simulink library "powerlib_extras"  (Simulink 6.0)
settings: Solver=ode45  SolverMode=SingleTasking  StartTime=0.0  StopTime=10.0  RelTol=1e-3
values from neighbouring files (symbols this model uses):
  Ts = get(handles.edit1,'string')    [powergui.m]
undefined symbols (not defined in the file or in its folder): Ac, Bc, Cc, Dc, Delay_discrete, dend, DiscIntNeverNeededParam, extra_sc, j, numd, test_alpha
libraries: powerlib2 x112, powerlib_extras x70, simulink_extras x25, simulink x12, powerlib_models x8
(part 4 of 9)

== system powerlib_extras/Control  Blocks/PWM Generator ==
  note: Pierre Giroux, Gilbert Sybille
      | Power System Laboratory, IREQ
      | Hydro-Quebec
  note: PWM Generator
  Signal(s) : Inport  Port=1  PortDimensions=Signal_PortWidth  LatchInput=off
  BL4 : Logic  Operator=NOT  Inputs=1
  BL5 : Logic  Operator=NOT  Inputs=1
  Constant : Constant  Value=Internal_Phase
  Constant1 : Constant  Value=Internal
  Data Type  Conversion : DataTypeConversion  Orientation=down  OutDataTypeMode=double  SaturateOnIntegerOverflow=on  RndMeth=Zero
  Data Type  Conversion1 : DataTypeConversion  OutDataTypeMode=boolean  SaturateOnIntegerOverflow=on  RndMeth=Zero
  Data Type  Conversion2 : DataTypeConversion  OutDataTypeMode=boolean  SaturateOnIntegerOverflow=on  RndMeth=Zero
  Gain : Gain  Gain=2*pi*Freq  SaturateOnIntegerOverflow=on
  Gain2 : Gain  Gain=pi/180  SaturateOnIntegerOverflow=on
  Gain3 : Gain  Gain=-1  SaturateOnIntegerOverflow=on
  Mux : Mux  Inputs=2
  Mux1 : Mux  Inputs=2
  Mux2 : Mux  Inputs=2
  Product : Product  SaturateOnIntegerOverflow=on  InputSameDT=on
  Relational Operator : RelationalOperator  InputSameDT=on
  Relational Operator1 : RelationalOperator  InputSameDT=on
  Select1A : Selector  Elements=Select1_Elements  InputPortWidth=Select1_PortWidth
  Select1B : Selector  Elements=Select1_Elements  InputPortWidth=Select1_PortWidth
  Select3 : Selector  Elements=Select3_Elements  InputPortWidth=Select3_PortWidth
  Sum : Sum  Inputs=+++  SaturateOnIntegerOverflow=on  InputSameDT=on
  Switch : Switch  Threshold=0.5  InputSameDT=on
  Triangle : simulink/Sources/Repeating Sequence  rep_seq_t=[0 1/Fc/4 3/Fc/4 1/Fc]  rep_seq_y=[0 -1 1 0]
  Trigonometric Function : Trigonometry
  m3 : Constant  Value=Phase
  m4 : Constant  Value=mIndex
  t : Clock
      settings: Decimation=10
  Pulses : Outport
  wires:
  Triangle/1 -> Relational Operator/2, Relational Operator1/2
  Switch/1 -> Relational Operator/1, Gain3/1
  Mux2/1 -> Select3/1
  Select1B/1 -> Mux2/2
  Select1A/1 -> Mux2/1
  Mux1/1 -> Select1B/1
  Mux/1 -> Select1A/1
  BL5/1 -> Mux1/2
  BL4/1 -> Mux/2
  Gain3/1 -> Relational Operator1/1
  Product/1 -> Switch/1
  Constant1/1 -> Switch/2
  Signal(s)/1 -> Switch/3
  Trigonometric Function/1 -> Product/2
  Sum/1 -> Trigonometric Function/1
  m4/1 -> Product/1
  Constant/1 -> Sum/3
  m3/1 -> Gain2/1
  Gain2/1 -> Sum/2
  Gain/1 -> Sum/1
  t/1 -> Gain/1
  Select3/1 -> Data Type  Conversion/1
  Data Type  Conversion/1 -> Pulses/1
  Relational Operator/1 -> Data Type  Conversion1/1
  Data Type  Conversion1/1 -> BL4/1, Mux/1
  Relational Operator1/1 -> Data Type  Conversion2/1
  Data Type  Conversion2/1 -> BL5/1, Mux1/1

== system powerlib_extras/Control  Blocks/Sample & Hold ==
  note: Sample and Hold
  note: Silvano Casoria
      | Power System Simulation Laboratory
      | IREQ, Hydro-Quebc
  In : Inport  Port=1  LatchInput=off
  S : Inport  Port=2  LatchInput=off
  IC=ic : Memory  Orientation=left  X0=ic  InheritSampleTime=on
  Switch : Switch  Threshold=0.5  SaturateOnIntegerOverflow=on  InputSameDT=on
  "   " : Outport  InitialOutput=0
  wires:
  Switch/1 -> "   "/1, IC=ic/1
  IC=ic/1 -> Switch/3
  In/1 -> Switch/1
  S/1 -> Switch/2

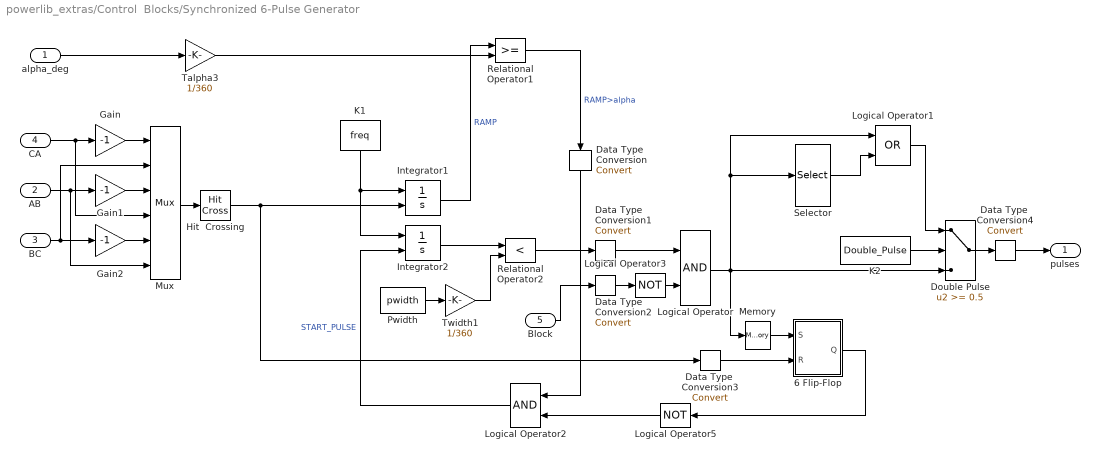
== system powerlib_extras/Control  Blocks/Synchronized 6-Pulse Generator ==
  alpha_deg : Inport  Port=1  LatchInput=off
  AB : Inport  Port=2  LatchInput=off
  BC : Inport  Port=3  LatchInput=off
  CA : Inport  Port=4  LatchInput=off
  Block : Inport  Port=5  LatchInput=off
  6 Flip-Flop : Subsystem
  Data Type  Conversion : DataTypeConversion  Orientation=down  OutDataTypeMode=boolean  SaturateOnIntegerOverflow=on  RndMeth=Zero
  Data Type  Conversion1 : DataTypeConversion  OutDataTypeMode=boolean  SaturateOnIntegerOverflow=on  RndMeth=Zero
  Data Type  Conversion2 : DataTypeConversion  OutDataTypeMode=boolean  SaturateOnIntegerOverflow=on  RndMeth=Zero
  Data Type  Conversion3 : DataTypeConversion  OutDataTypeMode=boolean  SaturateOnIntegerOverflow=on  RndMeth=Zero
  Data Type  Conversion4 : DataTypeConversion  OutDataTypeMode=double  SaturateOnIntegerOverflow=on  RndMeth=Zero
  Double Pulse : Switch  Threshold=0.5  InputSameDT=on
  Gain : Gain  Gain=-1  SaturateOnIntegerOverflow=on
  Gain1 : Gain  Gain=-1  SaturateOnIntegerOverflow=on
  Gain2 : Gain  Gain=-1  SaturateOnIntegerOverflow=on
  Hit  Crossing : HitCross  HitCrossingDirection=rising
  Integrator1 : Integrator  ExternalReset=rising
  Integrator2 : Integrator  ExternalReset=rising
  K1 : Constant  Orientation=down  Value=freq
  K2 : Constant  Value=Double_Pulse
  Logical Operator : Logic
  Logical Operator1 : Logic  Operator=OR
  Logical Operator2 : Logic  Orientation=left
  Logical Operator3 : Logic  Operator=NOT  Inputs=1
  Logical Operator5 : Logic  Orientation=left  Operator=NOT  Inputs=1
  Memory : Memory
  Mux : Mux  Inputs=6
  Pwidth : Constant  Value=pwidth
  Relational Operator1 : RelationalOperator  InputSameDT=on
  Relational Operator2 : RelationalOperator  Operator=<  InputSameDT=on
  Selector : Selector  Elements=[2 3 4 5 6 1 ]  InputPortWidth=6
  Talpha3 : Gain  Gain=1/360  SaturateOnIntegerOverflow=on
  Twidth1 : Gain  Gain=1/360  SaturateOnIntegerOverflow=on
  pulses : Outport  InitialOutput=0
  wires:
  alpha_deg/1 -> Talpha3/1
  Gain/1 -> Mux/1
  Gain1/1 -> Mux/3
  Gain2/1 -> Mux/5
  BC/1 -> Gain2/1, Mux/2
  CA/1 -> Gain/1, Mux/4
  AB/1 -> Gain1/1, Mux/6
  Mux/1 -> Hit  Crossing/1
  K1/1 -> Integrator1/1, Integrator2/1
  Pwidth/1 -> Twidth1/1
  Hit  Crossing/1 -> Integrator1/2, Data Type  Conversion3/1
  Logical Operator5/1 -> Logical Operator2/2
  Logical Operator2/1 -> Integrator2/2  "START_PULSE"
  6 Flip-Flop/1(Q) -> Logical Operator5/1
  Logical Operator3/1 -> Logical Operator/2
  Twidth1/1 -> Relational Operator2/2
  Integrator2/1 -> Relational Operator2/1
  Talpha3/1 -> Relational Operator1/2
  Integrator1/1 -> Relational Operator1/1  "RAMP"
  Memory/1 -> 6 Flip-Flop/1(S)
  K2/1 -> Double Pulse/2
  Logical Operator/1 -> Memory/1, Selector/1, Logical Operator1/1, Double Pulse/3
  Selector/1 -> Logical Operator1/2
  Relational Operator1/1 -> Data Type  Conversion/1  "RAMP>alpha"
  Data Type  Conversion/1 -> Logical Operator2/1
  Relational Operator2/1 -> Data Type  Conversion1/1
  Data Type  Conversion1/1 -> Logical Operator/1
  Block/1 -> Data Type  Conversion2/1
  Data Type  Conversion2/1 -> Logical Operator3/1
  Data Type  Conversion3/1 -> 6 Flip-Flop/2(R)
  Logical Operator1/1 -> Double Pulse/1
  Double Pulse/1 -> Data Type  Conversion4/1
  Data Type  Conversion4/1 -> pulses/1

== system powerlib_extras/Control  Blocks/Timer ==
  Clock : Clock
      settings: Decimation=10
  Derivative : Derivative
  Hit  Crossing : HitCross  ShowOutputPort=off
  Look-Up Table : Lookup  DialogController=Simulink.DDGSource  InputValues=tv  OutputValues=opv  SaturateOnIntegerOverflow=on
  Out : Outport
  wires:
  Derivative/1 -> Hit  Crossing/1
  Look-Up Table/1 -> Derivative/1, Out/1
  Clock/1 -> Look-Up Table/1

== system powerlib_extras/Discrete Measurements/Discrete PLL-Driven  Fundamental Value ==
  note: Pierre Giroux, Gilbert Sybille
      | Power System Simulation Laboratory
      | IREQ, Hydro-Quebc
  note: Discrete PLL-Driven Fundamental Value
  Freq : Inport  Port=1  LatchInput=off
  Sin_Cos : Inport  Port=2  PortDimensions=2  LatchInput=off
  In : Inport  Port=3  LatchInput=off
  Cartesian to Polar : simulink_extras/Transformations/Cartesian to Polar
  Demux : Demux  Outputs=2
  Discrete Variable Frequency Mean value : powerlib_extras/Discrete Measurements/Discrete Variable Frequency Mean value  Finit=Finit  Fmin=Fmin  Vinit=Real_Init  Ts=Ts
  Discrete Variable Frequency Mean value1 : powerlib_extras/Discrete Measurements/Discrete Variable Frequency Mean value  Finit=Finit  Fmin=Fmin  Vinit=Imag_Init  Ts=Ts
  Gain1 : Gain  Gain=2  SaturateOnIntegerOverflow=on
  Product : Product  SaturateOnIntegerOverflow=on  InputSameDT=on
  Rad->Deg. : Gain  Gain=180/pi  SaturateOnIntegerOverflow=on
  Mag : Outport
  Phase : Outport  Port=2
  wires:
  In/1 -> Product/1
  Sin_Cos/1 -> Gain1/1
  Freq/1 -> Discrete Variable Frequency Mean value/1, Discrete Variable Frequency Mean value1/1
  Demux/2 -> Discrete Variable Frequency Mean value1/2
  Product/1 -> Demux/1
  Gain1/1 -> Product/2
  Demux/1 -> Discrete Variable Frequency Mean value/2
  Rad->Deg./1 -> Phase/1
  Cartesian to Polar/1 -> Mag/1
  Cartesian to Polar/2 -> Rad->Deg./1
  Discrete Variable Frequency Mean value/1 -> Cartesian to Polar/1  "Real"
  Discrete Variable Frequency Mean value1/1 -> Cartesian to Polar/2  "Imag"

== system powerlib_extras/Discrete Measurements/Discrete Variable Frequency Mean value ==
  note: Variable frequency - Discrete Mean Value
  note: Pierre Giroux, Gilbert Sybille, Richard Gagnon
      | Power System Simulation Laboratory
      | IREQ, Hydro-Quebc
  note: link disabled
  Freq : Inport  Port=1  PortDimensions=1  LatchInput=off
  In : Inport  Port=2  PortDimensions=1  LatchInput=off
  Constant : Constant  Value=Vinit
  Correction subsystem : Subsystem
  Discrete Variable Transport Delay : Subsystem  AncestorBlock=|  mask(Discrete variable transport delay){MaxDelay=MaxDelay, InitialValue=0, Ts=Ts}
      | powerlib_extras/Discrete 
      | Control Blocks/Discrete Variable
      | Transport Delay
      mask prompts: MaxDelay "Maximum delay (s):"; InitialValue "Initial input:"; Ts "Sample time:"
      mask help:
      | Apply a delay to the first input (In) signal.
      | The second input (D) specifies the delay time.
  Gain : Gain  Gain=Ts  SaturateOnIntegerOverflow=on
  Integ4 : DiscreteIntegrator  IntegratorMethod=Integration: Trapezoidal  SampleTime=Ts  ICPrevOutput=DiscIntNeverNeededParam  ICPrevScaledInput=DiscIntNeverNeededParam
  Number of samples per cycle : Fcn  Expr=1/u[1]/Ts
  Product : Product  SaturateOnIntegerOverflow=on  InputSameDT=on
  Rounding Function : Rounding  Operator=ceil
  Step : Step  Time=1/Finit  SampleTime=Ts
  Sum5 : Sum  SaturateOnIntegerOverflow=on  InputSameDT=on
  Sum7 : Sum  Inputs=-+  SaturateOnIntegerOverflow=on  InputSameDT=on
  Switch : Switch  Threshold=0.5  InputSameDT=on
  To avoid division by zero : Saturate  Orientation=down  UpperLimit=1e6  LowerLimit=1e-6
  Mean : Outport
  wires:
  Step/1 -> Switch/2
  Correction subsystem/1(Out) -> Sum5/2
  To avoid division by zero/1 -> Number of samples per cycle/1  "Freq"
  Switch/1 -> Mean/1
  Constant/1 -> Switch/3
  Sum5/1 -> Switch/1
  Number of samples per cycle/1 -> Correction subsystem/1(N), Rounding Function/1
  Rounding Function/1 -> Correction subsystem/2(F), Gain/1
  Gain/1 -> Discrete Variable Transport Delay/2(D)  "Delay"
  Freq/1 -> To avoid division by zero/1, Product/2  "Freq"
  Integ4/1 -> Sum7/2, Discrete Variable Transport Delay/1(In)
  Sum7/1 -> Product/1
  Discrete Variable Transport Delay/1(Out) -> Sum7/1
  Product/1 -> Sum5/1  "Mean value"
  In/1 -> Correction subsystem/3(In), Integ4/1  "In"

== system powerlib_extras/Discrete Measurements/Discrete  Active  & Reactive  Power ==
  note: Pierre Giroux, Gilbert Sybille
      | Power System Simulation Laboratory
      | IREQ, Hydro-Quebc
  note: Discrete Active & Reactive Power at fundamental frequency
  V : Inport  Port=1  LatchInput=off
  I : Inport  Port=2  LatchInput=off
  Deg->Rad : Gain  Gain=pi/180  SaturateOnIntegerOverflow=on
  Discrete  I_Fundamental : powerlib_extras/Discrete Measurements/Discrete  Fourier  Freq=Freq  n=1  Par_Init=Par_Iinit  Ts=Ts
  Discrete  V_Fundamental : powerlib_extras/Discrete Measurements/Discrete  Fourier  Freq=Freq  n=1  Par_Init=Par_Vinit  Ts=Ts
  Gain : Gain  Gain=1/2  SaturateOnIntegerOverflow=on
  Mux : Mux  Inputs=2
  Mux1 : Mux  Inputs=2
  Product : Product  SaturateOnIntegerOverflow=on  InputSameDT=on
  Product1 : Product  SaturateOnIntegerOverflow=on  InputSameDT=on
  Product2 : Product  SaturateOnIntegerOverflow=on  InputSameDT=on
  Sum : Sum  Inputs=+-  SaturateOnIntegerOverflow=on  InputSameDT=on
  Trigonometric Function : Trigonometry
  Trigonometric Function1 : Trigonometry  Operator=cos
  Mag_V_I : Outport
  P_Q : Outport  Port=2
  wires:
  V/1 -> Discrete  V_Fundamental/1
  I/1 -> Discrete  I_Fundamental/1
  Discrete  V_Fundamental/2 -> Sum/1
  Discrete  I_Fundamental/2 -> Sum/2
  Sum/1 -> Deg->Rad/1
  Deg->Rad/1 -> Trigonometric Function1/1, Trigonometric Function/1
  Trigonometric Function/1 -> Product2/2
  Product/1 -> Product1/1, Product2/1
  Trigonometric Function1/1 -> Product1/2
  Mux/1 -> Mag_V_I/1
  Discrete  V_Fundamental/1 -> Product/1, Mux/1
  Discrete  I_Fundamental/1 -> Product/2, Mux/2
  Product1/1 -> Mux1/1
  Product2/1 -> Mux1/2
  Mux1/1 -> Gain/1
  Gain/1 -> P_Q/1

== system powerlib_extras/Discrete Measurements/Discrete  Fourier ==
  note: Discrete Fourier
  note: Pierre Giroux, Gilbert Sybille
      | Power System Simulation Laboratory
      | IREQ, Hydro-Quebc
  In : Inport  Port=1  LatchInput=off
  Cartesian to Polar : simulink_extras/Transformations/Cartesian to Polar
  Demux : Demux  Outputs=2
  Discrete  Mean value1 : powerlib_extras/Discrete Measurements/Discrete  Mean value  Freq=Freq  Vinit=Real_Init  Ts=Ts
  Discrete  Mean value2 : powerlib_extras/Discrete Measurements/Discrete  Mean value  Freq=Freq  Vinit=Imag_Init  Ts=Ts
  Gain : Gain  Gain=2*pi*n*Freq  SaturateOnIntegerOverflow=on
  Gain1 : Gain  Gain=k  SaturateOnIntegerOverflow=on
  Mux : Mux  Inputs=2
  Product : Product  SaturateOnIntegerOverflow=on  InputSameDT=on
  Rad->Deg. : Gain  Gain=180/pi  SaturateOnIntegerOverflow=on
  Trigonometric Function : Trigonometry
  Trigonometric Function1 : Trigonometry  Operator=cos
  t : DigitalClock  SampleTime=Ts
  Mag : Outport
  Phase : Outport  Port=2
  wires:
  t/1 -> Gain/1
  Gain/1 -> Trigonometric Function/1, Trigonometric Function1/1
  Trigonometric Function/1 -> Mux/1
  Trigonometric Function1/1 -> Mux/2
  Mux/1 -> Gain1/1
  In/1 -> Product/1
  Gain1/1 -> Product/2
  Product/1 -> Demux/1
  Demux/1 -> Discrete  Mean value1/1
  Demux/2 -> Discrete  Mean value2/1
  Discrete  Mean value1/1 -> Cartesian to Polar/1  "Real"
  Discrete  Mean value2/1 -> Cartesian to Polar/2  "Imag"
  Cartesian to Polar/2 -> Rad->Deg./1
  Cartesian to Polar/1 -> Mag/1
  Rad->Deg./1 -> Phase/1

== system powerlib_extras/Discrete Measurements/Discrete  Mean value ==
  note: Discrete Mean Value
  note: Pierre Giroux, Gilbert Sybille
      | Power System Simulation Laboratory
      | IREQ, Hydro-Quebc
  In : Inport  Port=1  LatchInput=off
  Constant : Constant  Value=Vinit
  Discrete Variable Transport Delay : powerlib_extras/Discrete  Control Blocks/Discrete Variable Transport Delay  MaxDelay=Delay+Ts  InitialValue=0  Ts=Ts
  Gain : Gain  Gain=K1  SaturateOnIntegerOverflow=on
  Gain1 : Gain  Gain=K2  SaturateOnIntegerOverflow=on
  Integ4 : DiscreteIntegrator  IntegratorMethod=Integration: Trapezoidal  SampleTime=Ts  ICPrevOutput=DiscIntNeverNeededParam  ICPrevScaledInput=DiscIntNeverNeededParam
  K1 : Constant  Value=Delay
  K2 : Constant  Value=Freq
  Product : Product  SaturateOnIntegerOverflow=on  InputSameDT=on
  Step : Step  Time=1/Freq  SampleTime=Ts
  Sum1 : Sum  Inputs=+-  SaturateOnIntegerOverflow=on  InputSameDT=on
  Sum5 : Sum  SaturateOnIntegerOverflow=on  InputSameDT=on
  Sum7 : Sum  Inputs=-+  SaturateOnIntegerOverflow=on  InputSameDT=on
  Switch : Switch  Threshold=0.5  InputSameDT=on
  Unit Delay : UnitDelay  SampleTime=Ts
  Mean : Outport
  wires:
  Sum1/1 -> Sum5/2  "Correction"
  Gain/1 -> Sum1/2
  Unit Delay/1 -> Gain/1
  Gain1/1 -> Sum1/1
  K1/1 -> Discrete Variable Transport Delay/2
  Discrete Variable Transport Delay/1 -> Sum7/1
  Switch/1 -> Mean/1
  Constant/1 -> Switch/3
  Step/1 -> Switch/2
  Sum5/1 -> Switch/1
  In/1 -> Unit Delay/1, Gain1/1, Integ4/1  "In"
  K2/1 -> Product/2
  Integ4/1 -> Sum7/2, Discrete Variable Transport Delay/1
  Sum7/1 -> Product/1
  Product/1 -> Sum5/1  "Mean value"

== system powerlib_extras/Discrete Measurements/Discrete  RMS value ==
  note: Gilbert Sybille, Pierre Giroux
      | Power System Simulation Laboratory
      | IREQ, Hydro-Quebc
  note: Discrete RMS value
  In : Inport  Port=1  LatchInput=off
  Discrete  Mean value : powerlib_extras/Discrete Measurements/Discrete  Mean value  Freq=Freq  Vinit=Mag_Init*Mag_Init  Ts=Ts
  Math Function1 : Math  Operator=sqrt  SaturateOnIntegerOverflow=on
  Product : Product  SaturateOnIntegerOverflow=on  InputSameDT=on
  Saturation Ajout P.B pour eviter  sqrt(negatif) : Saturate  UpperLimit=Inf  LowerLimit=0
  RMS : Outport  InitialOutput=0
  wires:
  In/1 -> Product/2, Product/1
  Math Function1/1 -> RMS/1
  Product/1 -> Discrete  Mean value/1
  Discrete  Mean value/1 -> Saturation Ajout P.B pour eviter  sqrt(negatif)/1
  Saturation Ajout P.B pour eviter  sqrt(negatif)/1 -> Math Function1/1

== system powerlib_extras/Discrete Measurements/Discrete  Total  Harmonic Distorsion ==
  note: Pierre Giroux, Gilbert Sybille
      | Power System Simulation Laboratory
      | IREQ, Hydro-Quebc
  note: Discrete Total Harmonic Distortion (THD)
  note: THD= Uhrms /U1rms
  note: Urms = true rms value including harmonics
  note: Uhrms = rms value of harmonics = sqrt( U2^2 + U3^2 + U4^2....) = sqrt( Urms^2 -U1rms^2)
  note: U1rms = rms value of the fundamenrtal component
  note: where:
  note: THD= Uhrms /U1rms
  signal : Inport  Port=1  LatchInput=off
  Constant : Constant  Value=1e-6
  Discrete  Fourier : powerlib_extras/Discrete Measurements/Discrete  Fourier  Freq=Freq  n=1  Par_Init=[0 0]  Ts=Ts
  Discrete  RMS value : powerlib_extras/Discrete Measurements/Discrete  RMS value  Freq=Freq  Mag_Init=0  Ts=Ts
  Math Function2 : Math  Operator=sqrt  SaturateOnIntegerOverflow=on
  Product : Product  Inputs=*/  SaturateOnIntegerOverflow=on  InputSameDT=on
  Product1 : Product  SaturateOnIntegerOverflow=on  InputSameDT=on
  Product2 : Product  SaturateOnIntegerOverflow=on  InputSameDT=on
  Sum : Sum  Inputs=+-  SaturateOnIntegerOverflow=on  InputSameDT=on
  Sum1 : Sum  Inputs=+-  SaturateOnIntegerOverflow=on  InputSameDT=on
  Terminator : Terminator
  peak2rms : Gain  Gain=1/sqrt(2)  SaturateOnIntegerOverflow=on
  THD : Outport
  wires:
  Sum1/1 -> Product/2
  Constant/1 -> Sum1/2
  Discrete  RMS value/1 -> Product1/2, Product1/1  "Urms"
  signal/1 -> Discrete  Fourier/1, Discrete  RMS value/1
  Sum/1 -> Math Function2/1
  Product1/1 -> Sum/1
  Product2/1 -> Sum/2
  Math Function2/1 -> Product/1  "Uhrms"
  Product/1 -> THD/1
  Discrete  Fourier/1 -> peak2rms/1
  peak2rms/1 -> Product2/2, Sum1/1, Product2/1  "U1 rms"
  Discrete  Fourier/2 -> Terminator/1

== system powerlib_extras/Discrete Measurements/Discrete 3-phase PLL-Driven Positive-Sequence Fundamental Value ==
  note: Pierre Giroux, Gilbert Sybille
      | Power System Simulation Laboratory
      | IREQ, Hydro-Quebc
  note: Discrete 3-phase PLL-Driven Positive-Sequence Fundamental Value
  Freq : Inport  Port=1  LatchInput=off
  Sin_Cos : Inport  Port=2  PortDimensions=2  LatchInput=off
  abc : Inport  Port=3  PortDimensions=3  LatchInput=off
  Cartesian to Polar : simulink_extras/Transformations/Cartesian to Polar
  Demux : Demux  Outputs=3
  Discrete Variable Frequency Mean value : powerlib_extras/Discrete Measurements/Discrete Variable Frequency Mean value  Finit=Finit  Fmin=Fmin  Vinit=Real_Init  Ts=Ts
  Discrete Variable Frequency Mean value1 : powerlib_extras/Discrete Measurements/Discrete Variable Frequency Mean value  Finit=Finit  Fmin=Fmin  Vinit=Imag_Init  Ts=Ts
  Rad->Deg. : Gain  Gain=180/pi  SaturateOnIntegerOverflow=on
  Terminator : Terminator
  abc_to_dq0 Transformation : powerlib_extras/Measurements/abc_to_dq0 Transformation
  Mag : Outport
  Phase : Outport  Port=2
  wires:
  Sin_Cos/1 -> abc_to_dq0 Transformation/2
  Freq/1 -> Discrete Variable Frequency Mean value/1, Discrete Variable Frequency Mean value1/1
  Discrete Variable Frequency Mean value/1 -> Cartesian to Polar/1  "Real"
  Rad->Deg./1 -> Phase/1
  Discrete Variable Frequency Mean value1/1 -> Cartesian to Polar/2  "Real"
  Demux/2 -> Discrete Variable Frequency Mean value1/2
  Demux/1 -> Discrete Variable Frequency Mean value/2
  abc/1 -> abc_to_dq0 Transformation/1
  abc_to_dq0 Transformation/1 -> Demux/1
  Demux/3 -> Terminator/1
  Cartesian to Polar/1 -> Mag/1
  Cartesian to Polar/2 -> Rad->Deg./1

== system powerlib_extras/Discrete Measurements/Discrete 3-phase PLL-Driven  Positive-Sequence Active & Reactive Power ==
  note: Pierre Giroux, Gilbert Sybille
      | Power System Simulation Laboratory
      | IREQ, Hydro-Quebc
  note: Discrete 3-phase PLL-driven Positive-Sequence Active & Reactive Power
  Freq : Inport  Port=1  PortDimensions=1  LatchInput=off
  Sin_Cos : Inport  Port=2  PortDimensions=2  LatchInput=off
  Vabc : Inport  Port=3  PortDimensions=3  LatchInput=off
  Iabc : Inport  Port=4  PortDimensions=3  LatchInput=off
  Deg->Rad : Gain  Gain=pi/180  SaturateOnIntegerOverflow=on
  Discrete 3-phase PLL-Driven Positive-Sequence Fundamental Value : powerlib_extras/Discrete Measurements/Discrete 3-phase PLL-Driven Positive-Sequence Fundamental Value  Finit=Finit  Fmin=Fmin  Par_Init=Par_Vinit  Ts=Ts
  Discrete 3-phase PLL-Driven Positive-Sequence Fundamental Value1 : powerlib_extras/Discrete Measurements/Discrete 3-phase PLL-Driven Positive-Sequence Fundamental Value  Finit=Finit  Fmin=Fmin  Par_Init=Par_Iinit  Ts=Ts
  Gain1 : Gain  Gain=3/2  SaturateOnIntegerOverflow=on
  Mux2 : Mux  Inputs=2
  Mux3 : Mux  Inputs=2
  Product : Product  SaturateOnIntegerOverflow=on  InputSameDT=on
  Product1 : Product  SaturateOnIntegerOverflow=on  InputSameDT=on
  Product2 : Product  SaturateOnIntegerOverflow=on  InputSameDT=on
  Sum : Sum  Inputs=+-  SaturateOnIntegerOverflow=on  InputSameDT=on
  Trigonometric Function : Trigonometry
  Trigonometric Function1 : Trigonometry  Operator=cos
  Mag_V_I : Outport
  P_Q : Outport  Port=2
  wires:
  Iabc/1 -> Discrete 3-phase PLL-Driven Positive-Sequence Fundamental Value1/3
  Discrete 3-phase PLL-Driven Positive-Sequence Fundamental Value1/1 -> Product2/2, Mux3/2
  Product2/1 -> Product1/2, Product/1
  Gain1/1 -> P_Q/1
  Mux3/1 -> Mag_V_I/1
  Product1/1 -> Mux2/2
  Product/1 -> Mux2/1
  Mux2/1 -> Gain1/1
  Trigonometric Function/1 -> Product1/1
  Trigonometric Function1/1 -> Product/2
  Deg->Rad/1 -> Trigonometric Function/1, Trigonometric Function1/1
  Sum/1 -> Deg->Rad/1
  Discrete 3-phase PLL-Driven Positive-Sequence Fundamental Value1/2 -> Sum/2
  Discrete 3-phase PLL-Driven Positive-Sequence Fundamental Value/1 -> Product2/1, Mux3/1
  Discrete 3-phase PLL-Driven Positive-Sequence Fundamental Value/2 -> Sum/1
  Sin_Cos/1 -> Discrete 3-phase PLL-Driven Positive-Sequence Fundamental Value/2, Discrete 3-phase PLL-Driven Positive-Sequence Fundamental Value1/2
  Freq/1 -> Discrete 3-phase PLL-Driven Positive-Sequence Fundamental Value/1, Discrete 3-phase PLL-Driven Positive-Sequence Fundamental Value1/1
  Vabc/1 -> Discrete 3-phase PLL-Driven Positive-Sequence Fundamental Value/3

== system powerlib_extras/Discrete Measurements/Discrete 3-phase Positive-Sequence Fundamental Value ==
  note: Discrete Measurement - Positive-sequence Fundamental Value
  note: Pierre Giroux, Gilbert Sybille
      | Power System Simulation Laboratory
      | IREQ, Hydro-Quebc
  abc : Inport  Port=1  PortDimensions=3  LatchInput=off
  Cartesian to Polar : simulink_extras/Transformations/Cartesian to Polar
  Demux : Demux  Outputs=3
  Discrete  Mean value1 : powerlib_extras/Discrete Measurements/Discrete  Mean value  Freq=Freq  Vinit=Real_Init  Ts=Ts
  Discrete  Mean value2 : powerlib_extras/Discrete Measurements/Discrete  Mean value  Freq=Freq  Vinit=Imag_Init  Ts=Ts
  Gain : Gain  Gain=2*pi*Freq  SaturateOnIntegerOverflow=on
  Mux : Mux  Inputs=2
  Rad->Deg. : Gain  Gain=180/pi  SaturateOnIntegerOverflow=on
  Terminator : Terminator
  Trigonometric Function : Trigonometry
  Trigonometric Function1 : Trigonometry  Operator=cos
  abc_to_dq0 Transformation : powerlib_extras/Measurements/abc_to_dq0 Transformation
  t : DigitalClock  SampleTime=Ts
  Mag : Outport
  Phase : Outport  Port=2
  wires:
  Trigonometric Function1/1 -> Mux/2
  Trigonometric Function/1 -> Mux/1
  Demux/1 -> Discrete  Mean value1/1
  Demux/2 -> Discrete  Mean value2/1
  Demux/3 -> Terminator/1
  abc_to_dq0 Transformation/1 -> Demux/1
  Discrete  Mean value2/1 -> Cartesian to Polar/2  "Real"
  Rad->Deg./1 -> Phase/1
  Discrete  Mean value1/1 -> Cartesian to Polar/1  "Real"
  Mux/1 -> abc_to_dq0 Transformation/2
  abc/1 -> abc_to_dq0 Transformation/1
  t/1 -> Gain/1
  Gain/1 -> Trigonometric Function/1, Trigonometric Function1/1
  Cartesian to Polar/1 -> Mag/1
  Cartesian to Polar/2 -> Rad->Deg./1

== system powerlib_extras/Discrete Measurements/Discrete 3-phase Sequence Analyzer ==
  note: Discrete 3-phase Sequence Analyser
  note: Gilbert Sybille, Pierre Giroux
      | Power System Simulation Laboratory
      | IREQ, Hydro-Quebc
  note: Zero sequence :V0 = 1/3 * (Va + Vb + Vc )
  note: where a =exp(j *2pi/3) = 1 < + 120 deg.
  note: Positive sequence :V1 = 1/3 * (Va + a*Vb + a^2 *Vc )
  note: Negative sequence :V2 = 1/3 * (Va + a^2*Vb + a *Vc )
  abc : Inport  Port=1  LatchInput=off
  Complex to Magnitude-Angle : ComplexToMagnitudeAngle
  Constant : Constant  Value=PosOn
  Constant1 : Constant  Value=NegOn
  Constant2 : Constant  Value=ZeroOn
  Demux : Demux  Outputs=3
  Determine if pha20 are set to zero : Subsystem
  "Gain2 " : Gain  Gain=k  SaturateOnIntegerOverflow=on
  Mux : Mux  Inputs=3
  Mux1 : Mux  Inputs=3
  Neg. Seq. Computation : Subsystem  TreatAsAtomicUnit=on
  Phasor A : Subsystem  mask(Discrete Fourier ; Real Imag Outputs){Freq=Freq, Par_Init=[Mag_Init  Phase_Init], Ts=Ts}
      mask prompts: Freq "Fundamental frequency (Hz):"; Par_Init "Initial Input [Mag Phase(degrees)]"; Ts "Sample time:"
      mask init:
      | Real_Init=Par_Init(1)*cos(Par_Init(2)*pi/180);
      | Imag_Init=Par_Init(1)*sin(Par_Init(2)*pi/180);
  Phasor B : powerlib_extras/Discrete Measurements/Discrete 3-phase Sequence Analyzer/Phasor A  Freq=Freq  Par_Init="[Mag_Init  Phase_Init-120]"  Ts=Ts
  Phasor C : powerlib_extras/Discrete Measurements/Discrete 3-phase Sequence Analyzer/Phasor A  Freq=Freq  Par_Init="[Mag_Init  Phase_Init+120]"  Ts=Ts
  Pos. Seq. Computation : Subsystem  TreatAsAtomicUnit=on
  Selector : Selector  Elements=SelectElement  InputPortWidth=3
  Selector1 : Selector  Elements=SelectElement  InputPortWidth=3
  Zero Seq. Computation : Subsystem  TreatAsAtomicUnit=on
  cos(nwt) : Sin  Frequency=2*pi*n*Freq  Phase=pi/2  SampleTime=Ts
  rad->deg1 : Gain  Gain=180/pi  SaturateOnIntegerOverflow=on
  sin(nwt) : Sin  Frequency=2*pi*n*Freq  SampleTime=Ts
  Mag : Outport  InitialOutput=0
  Phase : Outport  Port=2  InitialOutput=0
  wires:
  Phasor C/1 -> Mux/3
  Phasor B/1 -> Mux/2
  Phasor A/1(Out) -> Mux/1
  "Gain2 "/1 -> Demux/1
  abc/1 -> "Gain2 "/1
  Demux/1 -> Phasor A/1(in)
  Demux/2 -> Phasor B/1
  Demux/3 -> Phasor C/1
  sin(nwt)/1 -> Phasor A/2(sin), Phasor B/2, Phasor C/2
  cos(nwt)/1 -> Phasor A/3(cos), Phasor B/3, Phasor C/3
  Mux/1 -> Pos. Seq. Computation/1(In), Neg. Seq. Computation/1(In), Zero Seq. Computation/1(In)
  Pos. Seq. Computation/1(Out) -> Mux1/1
  Neg. Seq. Computation/1(Out) -> Mux1/2
  Zero Seq. Computation/1(Out) -> Mux1/3
  Mux1/1 -> Complex to Magnitude-Angle/1
  Complex to Magnitude-Angle/1 -> Determine if pha20 are set to zero/1(Mag120), Selector/1
  Constant/1 -> Pos. Seq. Computation/Enable
  Constant2/1 -> Zero Seq. Computation/Enable
  Selector/1 -> Mag/1
  Determine if pha20 are set to zero/1(Pha120) -> Selector1/1
  Selector1/1 -> rad->deg1/1
  rad->deg1/1 -> Phase/1
  Constant1/1 -> Neg. Seq. Computation/Enable
  Complex to Magnitude-Angle/2 -> Determine if pha20 are set to zero/2(Pha120*)

== system powerlib_extras/Discrete Measurements/Discrete 3-phase Total Power ==
  note: Pierre Giroux, Gilbert Sybille
      | Power System Simulation Laboratory
      | IREQ, Hydro-Quebc
  note: Discrete 3-phase Total Power
  Vabc : Inport  Port=1  PortDimensions=3  LatchInput=off
  Iabc : Inport  Port=2  PortDimensions=3  LatchInput=off
  Discrete  Mean value : powerlib_extras/Discrete Measurements/Discrete  Mean value  Freq=Freq  Vinit=P_Init  Ts=Ts
  Product3 : Product  SaturateOnIntegerOverflow=on  InputSameDT=on
  Sum1 : Sum  Inputs=1  SaturateOnIntegerOverflow=on  InputSameDT=on
  Pinst : Outport
  Pmean : Outport  Port=2
  wires:
  Sum1/1 -> Discrete  Mean value/1, Pinst/1
  Discrete  Mean value/1 -> Pmean/1
  Iabc/1 -> Product3/2
  Product3/1 -> Sum1/1
  Vabc/1 -> Product3/1

== system powerlib_extras/Discrete Measurements/Discrete 3-phase  Positive-Sequence  Active & Reactive Power ==
  note: Discrete 3-phase Positive-Sequence Active & Reactive Power
  note: Pierre Giroux, Gilbert Sybille
      | Power System Simulation Laboratory
      | IREQ, Hydro-Quebc
  Vabc : Inport  Port=1  PortDimensions=3  LatchInput=off
  Iabc : Inport  Port=2  PortDimensions=3  LatchInput=off
  Deg->Rad : Gain  Gain=pi/180  SaturateOnIntegerOverflow=on
  Discrete 3-phase Positive-Sequence Fundamental Value (I) : powerlib_extras/Discrete Measurements/Discrete 3-phase Positive-Sequence Fundamental Value  Freq=Freq  Par_Init=Par_Iinit  Ts=Ts
  Discrete 3-phase Positive-Sequence Fundamental Value (V) : powerlib_extras/Discrete Measurements/Discrete 3-phase Positive-Sequence Fundamental Value  Freq=Freq  Par_Init=Par_Vinit  Ts=Ts
  Gain1 : Gain  Gain=3/2  SaturateOnIntegerOverflow=on
  Mux2 : Mux  Inputs=2
  Mux3 : Mux  Inputs=2
  Product : Product  SaturateOnIntegerOverflow=on  InputSameDT=on
  Product1 : Product  SaturateOnIntegerOverflow=on  InputSameDT=on
  Product2 : Product  SaturateOnIntegerOverflow=on  InputSameDT=on
  Sum : Sum  Inputs=+-  SaturateOnIntegerOverflow=on  InputSameDT=on
  Trigonometric Function : Trigonometry
  Trigonometric Function1 : Trigonometry  Operator=cos
  Mag_V_I : Outport
  P_Q : Outport  Port=2
  wires:
  Vabc/1 -> Discrete 3-phase Positive-Sequence Fundamental Value (V)/1
  Iabc/1 -> Discrete 3-phase Positive-Sequence Fundamental Value (I)/1
  Discrete 3-phase Positive-Sequence Fundamental Value (V)/2 -> Sum/1
  Discrete 3-phase Positive-Sequence Fundamental Value (I)/2 -> Sum/2
  Sum/1 -> Deg->Rad/1
  Deg->Rad/1 -> Trigonometric Function1/1, Trigonometric Function/1
  Trigonometric Function1/1 -> Product/2
  Trigonometric Function/1 -> Product1/1
  Mux2/1 -> Gain1/1
  Product/1 -> Mux2/1
  Product1/1 -> Mux2/2
  Mux3/1 -> Mag_V_I/1
  Gain1/1 -> P_Q/1
  Product2/1 -> Product/1, Product1/2
  Discrete 3-phase Positive-Sequence Fundamental Value (V)/1 -> Mux3/1, Product2/1
  Discrete 3-phase Positive-Sequence Fundamental Value (I)/1 -> Mux3/2, Product2/2

== system powerlib_extras/Discrete Measurements/FFT ==
  note: P.Dahler
      | ABB Industrie AG
      | Turgi, Switzerland
  f(k) : Inport  Port=1  LatchInput=off
  Constant1 : Constant  Value=base
  Constant2 : Constant  Value=nDec*ones(1,Nsig)
  Constant3 : Constant  Value=mask
  Constant4 : Constant  Value=figure_N*ones(1,Nsig)
  Discrete Shift Register : powerlib_extras/Discrete  Control Blocks/Discrete Shift Register  NSamples=Navg  InitialValue=0  Ts=Ts
  MATLAB Fcn executing and plotting FFT : MATLABFcn  MATLABFcn=fft_function  OutputDimensions="[ceil(Navg/2) + 5  Nsig]"  Output1D=off
  Matrix Concatenation1 : simulink/Math Operations/Matrix Concatenation  numInports=5  catMethod=Vertical
  Reshape : simulink/Math Operations/Reshape  OutputDimensionality=Customize  OutputDimensions=[Navg,Nsig]
  Reshape{1..4} (4 alike) : simulink/Math Operations/Reshape  OutputDimensionality=Customize  OutputDimensions=[1 Nsig]
  Selector : Selector  InputType=Matrix  Elements=[1:ceil(Navg/2)]  Rows=1:ceil(Navg/2)  Columns=1:Nsig  InputPortWidth=ceil(Navg/2) + 5
  Selector1 : Selector  InputType=Matrix  Elements=[1:ceil(Navg/2)]  Rows=ceil(Navg/2)+1 : ceil(Navg/2)+5  Columns=1:Nsig  InputPortWidth=ceil(Navg/2) + 5
  TsFFT1 : ZeroOrderHold  SampleTime=TsFFT
  F(n) : Outport
  RMS : Outport  Port=2
  wires:
  Reshape4/1 -> Matrix Concatenation1/5
  Reshape/1 -> TsFFT1/1
  TsFFT1/1 -> Matrix Concatenation1/1
  Reshape3/1 -> Matrix Concatenation1/4
  Reshape2/1 -> Matrix Concatenation1/3
  Reshape1/1 -> Matrix Concatenation1/2
  Constant4/1 -> Reshape4/1
  Constant3/1 -> Reshape3/1
  Constant2/1 -> Reshape2/1
  Constant1/1 -> Reshape1/1
  Matrix Concatenation1/1 -> MATLAB Fcn executing and plotting FFT/1
  MATLAB Fcn executing and plotting FFT/1 -> Selector1/1, Selector/1
  Selector/1 -> F(n)/1
  Selector1/1 -> RMS/1
  f(k)/1 -> Discrete Shift Register/1
  Discrete Shift Register/1 -> Reshape/1

== system powerlib_extras/Discrete  Control Blocks/Discrete 1-phase PLL ==
  note: Discrete 1-phase PLL
  note: Pierre Giroux, Gilbert Sybille
      | Power System Laboratory, IREQ
      | Hydro-Quebec
  note: Note: sin( a ) * cos( b )= 1/2 * sin( a+b ) + 1/2 * sin(a-b)
  V(pu) : Inport  Port=1  LatchInput=off
  Constant4 : Constant  Value=2*pi
  Discrete PI Controller : powerlib_extras/Discrete  Control Blocks/Discrete PI Controller  Kp=Kp  Ki=Ki  Par_Limits="[1.25  0.75]*2*pi*Finit"  Init=2*pi*Finit  Ts=Ts
  Discrete Rate Limiter : powerlib_extras/Discrete  Control Blocks/Discrete Rate Limiter  R=12  F=-12  Vinit=Finit  Ts=Ts
  Discrete Variable Frequency Mean value : powerlib_extras/Discrete Measurements/Discrete Variable Frequency Mean value  Finit=Finit  Fmin=Fmin  Vinit=0  Ts=Ts
  Discrete  2nd-Order Filter : powerlib_extras/Discrete  Control Blocks/Discrete  2nd-Order Filter  FilterType=Lowpass  Fo=25  Zeta=0.707  Ts=Ts  Initialize=on  Vac_Init="[0 0  Finit]"  Vdc_Init=Finit  PlotResponse=off  param1=[1 500 0.1]
  Discrete-Time Integrator : DiscreteIntegrator  InitialCondition=Phase_Init*pi/180  SampleTime=Ts  ICPrevOutput=DiscIntNeverNeededParam  ICPrevScaledInput=DiscIntNeverNeededParam
  Gain10 : Gain  Gain=1/2/pi  SaturateOnIntegerOverflow=on
  Math Function : Math  Operator=mod  SaturateOnIntegerOverflow=on
  Mux1 : Mux  Inputs=2
  Product1 : Product  SaturateOnIntegerOverflow=on  InputSameDT=on
  Trigonometric Function5 : Trigonometry  Operator=cos
  Trigonometric Function6 : Trigonometry
  Unit Delay1 : UnitDelay  X0=Finit  SampleTime=Ts
  Freq : Outport
  wt : Outport  Port=2
  Sin_Cos : Outport  Port=3
  wires:
  Trigonometric Function5/1 -> Product1/2, Mux1/2
  Trigonometric Function6/1 -> Mux1/1
  Math Function/1 -> wt/1, Trigonometric Function5/1, Trigonometric Function6/1
  Mux1/1 -> Sin_Cos/1
  Discrete Variable Frequency Mean value/1 -> Discrete PI Controller/1
  Product1/1 -> Discrete Variable Frequency Mean value/2
  Discrete-Time Integrator/1 -> Math Function/1
  Constant4/1 -> Math Function/2
  V(pu)/1 -> Product1/1
  Discrete PI Controller/1 -> Discrete-Time Integrator/1, Gain10/1  "W"
  Gain10/1 -> Discrete Rate Limiter/1
  Discrete Rate Limiter/1 -> Discrete  2nd-Order Filter/1
  Discrete  2nd-Order Filter/1 -> Unit Delay1/1
  Unit Delay1/1 -> Freq/1, Discrete Variable Frequency Mean value/1

== system powerlib_extras/Discrete  Control Blocks/Discrete 1st-Order Discrete Filter ==
  In : Inport  Port=1  LatchInput=off
  Discrete State-Space : DiscreteStateSpace  A=Ad  B=Bd  C=Cd  D=Dd  X0=x0d  SampleTime=Ts
  Out : Outport  InitialOutput=0
  wires:
  In/1 -> Discrete State-Space/1
  Discrete State-Space/1 -> Out/1

== system powerlib_extras/Discrete  Control Blocks/Discrete 1st-Order Filter ==
  In : Inport  Port=1  LatchInput=off
  Discrete State-Space : DiscreteStateSpace  A=Ad  B=Bd  C=Cd  D=Dd  X0=x0d  SampleTime=Ts
  Out : Outport  InitialOutput=0
  wires:
  Discrete State-Space/1 -> Out/1
  In/1 -> Discrete State-Space/1

== system powerlib_extras/Discrete  Control Blocks/Discrete 2nd-Order Variable-Tuned Filter ==
  note: 2nd Order Discrete
      | Variable Tuned Filter
  note: Pierre Giroux, Frederic Giguere
      | Power System Simulation Laboratory
      | IREQ, Hydro-Quebc
  note: Electrical representation of a 2nd order filter --> Series RLC
  note: VC/Vin --> Lowpass
  note: VL/Vin --> Highpass
  note: VR/Vin --> Bandpass
  note: (VL+VC)/Vin --> Bandstop (Notch)
  note: Correction factor
      | to achieve accurate "Fo"
      | for discrete filter
  Fo : Inport  Port=1  LatchInput=off
  In : Inport  Port=2  LatchInput=off
  Cor : Constant  Value=Correction
  Corrige1 : Constant  Value=Zeta
  Corrige2 : Constant  Value=FilterType
  Discrete-Time Integrator : DiscreteIntegrator  IntegratorMethod=Integration: Trapezoidal  InitialCondition=Iinit  SampleTime=Ts  ICPrevOutput=DiscIntNeverNeededParam  ICPrevScaledInput=DiscIntNeverNeededParam
  Discrete-Time Integrator1 : DiscreteIntegrator  IntegratorMethod=Integration: Trapezoidal  InitialCondition=VC  SampleTime=Ts  ICPrevOutput=DiscIntNeverNeededParam  ICPrevScaledInput=DiscIntNeverNeededParam
  Gain : Gain  Gain=2*pi  SaturateOnIntegerOverflow=on
  Gain1 : Gain  Gain=2  SaturateOnIntegerOverflow=on
  Multiport Switch : MultiPortSwitch  InputSameDT=on
  Predict1 : Subsystem
  Product : Product  Inputs=**  SaturateOnIntegerOverflow=on  InputSameDT=on
  Product1 : Product  Inputs=**  SaturateOnIntegerOverflow=on  InputSameDT=on
  Product2 : Product  Inputs=***  SaturateOnIntegerOverflow=on  InputSameDT=on
  Product3 : Product  Inputs=****  SaturateOnIntegerOverflow=on  InputSameDT=on
  Sum : Sum  Inputs=+--  SaturateOnIntegerOverflow=on  InputSameDT=on
  Sum1 : Sum  Inputs=+-  SaturateOnIntegerOverflow=on  InputSameDT=on
  Sum2 : Sum  SaturateOnIntegerOverflow=on  InputSameDT=on
  Unit Delay6 : UnitDelay  X0=VL  SampleTime=Ts
  Out : Outport
  wires:
  Product1/1 -> Product/1
  Gain/1 -> Product1/2, Product1/1, Product2/2
  Product/1 -> Discrete-Time Integrator1/1
  Fo/1 -> Sum1/1, Product3/1, Product3/2, Product3/3
  Cor/1 -> Product3/4
  Product3/1 -> Sum1/2
  Sum1/1 -> Gain/1
  In/1 -> Sum/1  "Vin"
  Discrete-Time Integrator1/1 -> Sum/3, Multiport Switch/2, Sum2/2  "VC"
  Product2/1 -> Sum/2, Multiport Switch/4  "VR"
  Corrige2/1 -> Multiport Switch/1
  Discrete-Time Integrator/1 -> Product2/3, Product/2  "I"
  Unit Delay6/1 -> Predict1/1(In)
  Predict1/1(Out) -> Discrete-Time Integrator/1
  Sum/1 -> Unit Delay6/1, Multiport Switch/3, Sum2/1  "VL"
  Sum2/1 -> Multiport Switch/5
  Multiport Switch/1 -> Out/1
  Corrige1/1 -> Gain1/1
  Gain1/1 -> Product2/1

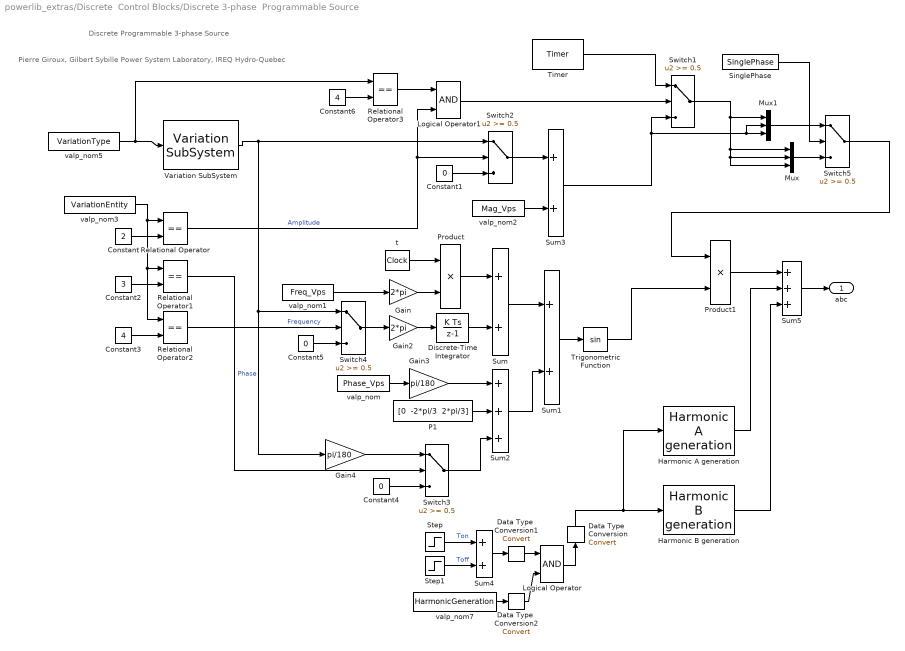
== system powerlib_extras/Discrete  Control Blocks/Discrete 3-phase  Programmable Source ==
  note: Discrete Programmable 3-phase Source
  note: Pierre Giroux, Gilbert Sybille
      | Power System Laboratory, IREQ
      | Hydro-Quebec
  Constant : Constant  Value=2
  Constant1 : Constant  Value=0
  Constant2 : Constant  Value=3
  Constant3 : Constant  Value=4
  Constant4 : Constant  Value=0
  Constant5 : Constant  Value=0
  Constant6 : Constant  Value=4
  Data Type  Conversion : DataTypeConversion  Orientation=up  OutDataTypeMode=double  SaturateOnIntegerOverflow=on  RndMeth=Zero
  Data Type  Conversion1 : DataTypeConversion  OutDataTypeMode=boolean  SaturateOnIntegerOverflow=on  RndMeth=Zero
  Data Type  Conversion2 : DataTypeConversion  OutDataTypeMode=boolean  SaturateOnIntegerOverflow=on  RndMeth=Zero
  Discrete-Time Integrator : DiscreteIntegrator  SampleTime=Ts  ICPrevOutput=DiscIntNeverNeededParam  ICPrevScaledInput=DiscIntNeverNeededParam
  Gain : Gain  Gain=2*pi  SaturateOnIntegerOverflow=on
  Gain2 : Gain  Gain=2*pi  SaturateOnIntegerOverflow=on
  Gain3 : Gain  Gain=pi/180  SaturateOnIntegerOverflow=on
  Gain4 : Gain  Gain=pi/180  SaturateOnIntegerOverflow=on
  Harmonic A generation : powerlib_models/Discrete/3_Phase_Prog_Source/Harmonic A generation  Freq_Vps=Freq_Vps  n_Harmo=n_HarmoA  Mag_Harmo=Mag_HarmoA  Phase_Harmo=Phase_HarmoA  Seq_Harmo=Seq_HarmoA  Ts=Ts
  Harmonic B generation : powerlib_models/Discrete/3_Phase_Prog_Source/Harmonic B generation  Freq_Vps=Freq_Vps  n_Harmo=n_HarmoB  Mag_Harmo=Mag_HarmoB  Phase_Harmo=Phase_HarmoB  Seq_Harmo=Seq_HarmoB  Ts=Ts
  Logical Operator : Logic
  Logical Operator1 : Logic
  Mux : Mux  Inputs=3
  Mux1 : Mux  Inputs=3
  P1 : Constant  Value="[0  -2*pi/3  2*pi/3]"
  Product : Product  SaturateOnIntegerOverflow=on  InputSameDT=on
  Product1 : Product  SaturateOnIntegerOverflow=on  InputSameDT=on
  Relational Operator{,1..3} (4 alike) : RelationalOperator  Operator===  InputSameDT=on
  SinglePhase : Constant  Value=SinglePhase
  Step : Step  Time=Ton_Harmo  SampleTime=Ts
  Step1 : Step  Time=Toff_Harmo  After=-1  SampleTime=Ts
  Sum{,1,3..4} (4 alike) : Sum  SaturateOnIntegerOverflow=on  InputSameDT=on
  Sum2 : Sum  Inputs=+++  SaturateOnIntegerOverflow=on  InputSameDT=on
  Sum5 : Sum  Inputs=+++  SaturateOnIntegerOverflow=on  InputSameDT=on
  Switch{1..5} (5 alike) : Switch  Threshold=0.5  InputSameDT=on
  Timer : powerlib_models/Discrete/3_Phase_Prog_Source/Timer  t=Xtime  e=Yampli  Ts=Ts
  Trigonometric Function : Trigonometry
  Variation SubSystem : powerlib_models/Discrete/3_Phase_Prog_Source/Variation SubSystem  VariationStep=VariationStep  VariationRate=VariationRate  VariationFreq=VariationFreq  VariationMag=VariationMag  Ton_Variation=Ton_Variation  Toff_Variation=Toff_Variation  Ts=Ts
  t : DigitalClock  SampleTime=Ts
  valp_nom : Constant  Value=Phase_Vps
  valp_nom1 : Constant  Value=Freq_Vps
  valp_nom2 : Constant  Value=Mag_Vps
  valp_nom3 : Constant  Value=VariationEntity
  valp_nom5 : Constant  Value=VariationType
  valp_nom7 : Constant  Value=HarmonicGeneration
  abc : Outport  InitialOutput=0
  wires:
  Data Type  Conversion2/1 -> Logical Operator/2
  valp_nom7/1 -> Data Type  Conversion2/1
  Data Type  Conversion1/1 -> Logical Operator/1
  Sum4/1 -> Data Type  Conversion1/1
  Data Type  Conversion/1 -> Harmonic B generation/1, Harmonic A generation/1
  Logical Operator/1 -> Data Type  Conversion/1
  Product/1 -> Sum/1
  Gain/1 -> Product/2
  t/1 -> Product/1
  Sum/1 -> Sum1/1
  Sum1/1 -> Trigonometric Function/1
  Gain2/1 -> Discrete-Time Integrator/1
  Discrete-Time Integrator/1 -> Sum/2
  P1/1 -> Sum2/2
  Trigonometric Function/1 -> Product1/2
  Gain3/1 -> Sum2/1
  valp_nom/1 -> Gain3/1
  valp_nom1/1 -> Gain/1
  Product1/1 -> Sum5/1
  Switch2/1 -> Sum3/1
  Constant1/1 -> Switch2/3
  Sum2/1 -> Sum1/2
  valp_nom2/1 -> Sum3/2
  Relational Operator/1 -> Switch2/2, Logical Operator1/2  "Amplitude"
  valp_nom5/1 -> Variation SubSystem/1, Relational Operator3/1
  Switch3/1 -> Sum2/3
  Constant4/1 -> Switch3/3
  Relational Operator1/1 -> Switch3/2  "Phase"
  Variation SubSystem/1 -> Switch2/1, Switch4/1, Gain4/1
  Switch4/1 -> Gain2/1
  Relational Operator2/1 -> Switch4/2  "Frequency"
  Constant/1 -> Relational Operator/2
  valp_nom3/1 -> Relational Operator/1, Relational Operator2/1, Relational Operator1/1
  Constant2/1 -> Relational Operator1/2
  Constant3/1 -> Relational Operator2/2
  Constant5/1 -> Switch4/3
  Harmonic A generation/1 -> Sum5/2
  Sum5/1 -> abc/1
  Step/1 -> Sum4/1  "Ton"
  Step1/1 -> Sum4/2  "Toff"
  Harmonic B generation/1 -> Sum5/3
  Gain4/1 -> Switch3/1
  Constant6/1 -> Relational Operator3/2
  Sum3/1 -> Switch1/3, Mux1/3, Mux1/2
  Timer/1 -> Switch1/1
  Mux1/1 -> Switch5/1
  SinglePhase/1 -> Switch5/2
  Mux/1 -> Switch5/3
  Switch1/1 -> Mux/1, Mux/2, Mux/3, Mux1/1
  Switch5/1 -> Product1/1
  Relational Operator3/1 -> Logical Operator1/1
  Logical Operator1/1 -> Switch1/2

== system powerlib_extras/Discrete  Control Blocks/Discrete 3-phase PLL ==
  note: Discrete 3-phase PLL
  note: Pierre Giroux, Gilbert Sybille
      | Power System Laboratory, IREQ
      | Hydro-Quebec
  Vabc (pu) : Inport  Port=1  PortDimensions=3  LatchInput=off
  Constant4 : Constant  Value=2*pi
  Discrete PI Controller : powerlib_extras/Discrete  Control Blocks/Discrete PI Controller  Kp=Kp  Ki=Ki  Par_Limits=2*pi*Finit*[1.25 0.75]  Init=2*pi*Finit  Ts=Ts
  Discrete Rate Limiter : powerlib_extras/Discrete  Control Blocks/Discrete Rate Limiter  R=12  F=-12  Vinit=Finit  Ts=Ts
  Discrete Variable Frequency Mean value : powerlib_extras/Discrete Measurements/Discrete Variable Frequency Mean value  Finit=Finit  Fmin=Fmin  Vinit=0  Ts=Ts
  Discrete  2nd-Order Filter : powerlib_extras/Discrete  Control Blocks/Discrete  2nd-Order Filter  FilterType=Lowpass  Fo=25  Zeta=0.707  Ts=Ts  Initialize=on  Vac_Init=[0 0 Finit]  Vdc_Init=Finit  PlotResponse=off  param1=[1 500 0.1]
  Discrete-Time Integrator : DiscreteIntegrator  InitialCondition=Phase_Init*pi/180  SampleTime=Ts  ICPrevOutput=DiscIntNeverNeededParam  ICPrevScaledInput=DiscIntNeverNeededParam
  Gain10 : Gain  Gain=1/2/pi  SaturateOnIntegerOverflow=on
  Math Function : Math  Operator=mod  SaturateOnIntegerOverflow=on
  Mux2 : Mux  Inputs=2
  Selector : Selector  Elements=2  InputPortWidth=3
  Trigonometric Function : Trigonometry
  Trigonometric Function2 : Trigonometry  Operator=cos
  Unit Delay : UnitDelay  X0=Finit  SampleTime=Ts
  abc_to_dq0 Transformation : powerlib_extras/Measurements/abc_to_dq0 Transformation
  Freq : Outport
  wt : Outport  Port=2
  Sin_Cos : Outport  Port=3
  wires:
  Discrete Variable Frequency Mean value/1 -> Discrete PI Controller/1
  Vabc (pu)/1 -> abc_to_dq0 Transformation/1
  abc_to_dq0 Transformation/1 -> Selector/1
  Constant4/1 -> Math Function/2
  Discrete-Time Integrator/1 -> Math Function/1
  Math Function/1 -> Trigonometric Function/1, Trigonometric Function2/1, wt/1
  Trigonometric Function/1 -> Mux2/1
  Trigonometric Function2/1 -> Mux2/2
  Mux2/1 -> abc_to_dq0 Transformation/2, Sin_Cos/1
  Discrete PI Controller/1 -> Discrete-Time Integrator/1, Gain10/1  "W"
  Gain10/1 -> Discrete Rate Limiter/1
  Discrete Rate Limiter/1 -> Discrete  2nd-Order Filter/1
  Unit Delay/1 -> Freq/1, Discrete Variable Frequency Mean value/1
  Discrete  2nd-Order Filter/1 -> Unit Delay/1
  Selector/1 -> Discrete Variable Frequency Mean value/2  "Vq"

== system powerlib_extras/Discrete  Control Blocks/Discrete Bistable ==
  note: Discrete Bistable Flip-Flop with priority to Set or Reset
  note: Silvano Casoria
      | Power System Simulation Laboratory
      | IREQ, Hydro-Quebc
  S : Inport  Port=1  LatchInput=off
  R : Inport  Port=2  LatchInput=off
  Constant : Constant
  Constant2 : Constant  Value=priority
  Data Type Conversion1 : DataTypeConversion  OutDataTypeMode=boolean  SaturateOnIntegerOverflow=on  RndMeth=Zero
  Data Type Conversion2 : DataTypeConversion  OutDataTypeMode=boolean  SaturateOnIntegerOverflow=on  RndMeth=Zero
  Logical Operator1 : Logic  Operator=OR
  Logical Operator2 : Logic  Operator=NOT  Inputs=1
  Logical Operator3 : Logic  Operator=OR
  RESET Priority : Subsystem  TreatAsAtomicUnit=on
  Relational Operator1 : RelationalOperator  Operator=>  InputSameDT=on
  SET  Priority : Subsystem  TreatAsAtomicUnit=on
  Q : Outport  InitialOutput=0
  !Q : Outport  Port=2  InitialOutput=1
  wires:
  R/1 -> Data Type Conversion1/1
  S/1 -> Data Type Conversion2/1
  Data Type Conversion2/1 -> RESET Priority/1(S), SET  Priority/1(S)
  Data Type Conversion1/1 -> RESET Priority/2(R), SET  Priority/2(R)
  Logical Operator2/1 -> RESET Priority/Enable
  Constant2/1 -> Relational Operator1/1
  Relational Operator1/1 -> Logical Operator2/1, SET  Priority/Enable
  Constant/1 -> Relational Operator1/2
  SET  Priority/1(Q) -> Logical Operator1/1
  Logical Operator1/1 -> Q/1
  SET  Priority/2(!Q) -> Logical Operator3/1
  Logical Operator3/1 -> !Q/1
  RESET Priority/1(Q) -> Logical Operator1/2
  RESET Priority/2(!Q) -> Logical Operator3/2

== system powerlib_extras/Discrete  Control Blocks/Discrete Edge Detector ==
  note: Edge or Slope Detector
  note: Silvano Casoria
      | Power System Simulation Laboratory
      | IREQ, Hydro-Quebc
  In : Inport  Port=1  LatchInput=off
  Constant1 : Constant  Value=model
  Demux : Demux  Outputs=2
  Logical Operator1 : Logic  Operator=OR
  Multiport Switch : MultiPortSwitch  Inputs=3  SaturateOnIntegerOverflow=on
  NEGATIVE Edge : Subsystem  AncestorBlock=extra_sc/Edge/POSITIVE Edge  TreatAsAtomicUnit=on
  POSITIVE Edge : Subsystem  AncestorBlock=extra_sc/Delay_discrete/OFF Delay  TreatAsAtomicUnit=on
  Unit Delay : UnitDelay  X0=ic  SampleTime=Ts
  either edge : Constant  Value=[1 1]
  neg. edge : Constant  Value=[0 1]
  pos. edge : Constant  Value=[1 0]
  Out : Outport
  wires:
  either edge/1 -> Multiport Switch/4
  Demux/2 -> NEGATIVE Edge/Enable
  Demux/1 -> POSITIVE Edge/Enable
  Multiport Switch/1 -> Demux/1
  Constant1/1 -> Multiport Switch/1
  neg. edge/1 -> Multiport Switch/3
  pos. edge/1 -> Multiport Switch/2
  In/1 -> Unit Delay/1, NEGATIVE Edge/1(IN), POSITIVE Edge/1(IN)
  Unit Delay/1 -> NEGATIVE Edge/2(IN previous), POSITIVE Edge/2(IN previous)
  POSITIVE Edge/1(OUT) -> Logical Operator1/1
  NEGATIVE Edge/1(OUT) -> Logical Operator1/2
  Logical Operator1/1 -> Out/1

== system powerlib_extras/Discrete  Control Blocks/Discrete Lead-Lag ==
  In1 : Inport  Port=1  LatchInput=off
  Discrete State-Space : DiscreteStateSpace  A=Ad  B=Bd  C=Cd  D=Dd  X0=x0d  SampleTime=Ts
  Out1 : Outport
  wires:
  In1/1 -> Discrete State-Space/1
  Discrete State-Space/1 -> Out1/1
